simulink model "Question_1"  (R2024b)
settings: Solver=VariableStepAuto  StartTime=0.0  StopTime=10.0  RelTol=1e-3
model workspace (MAT data in the model file):
  b1 = 50
  b2 = 70
  k1 = 400
  k2 = 600
  m = 100
settings Model: Creator=Sagar  LastModifiedBy=Sagar

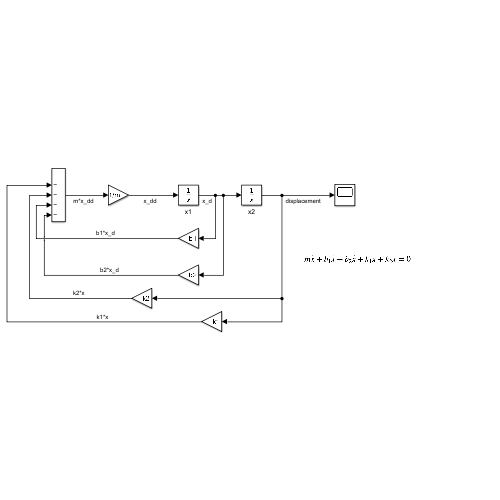
[thumbnail: Simulink's stored preview of the top-level diagram]
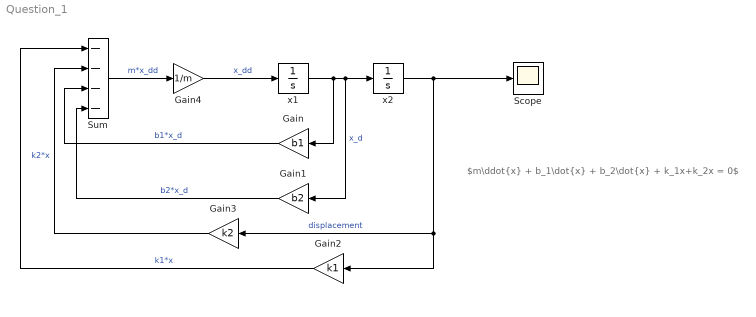
== system Question_1 ==
  note: $m\ddot{x} + b_1\dot{x} + b_2\dot{x} + k_1x+k_2x = 0$
  Gain : Gain  Gain=b1
  Gain1 : Gain  Gain=b2
  Gain2 : Gain  Gain=k1
  Gain3 : Gain  Gain=k2
  Gain4 : Gain  Gain=1/m
  Scope : Scope
  Sum : Sum  Inputs=|----
  x1 : Integrator
  x2 : Integrator  InitialCondition=0.8
  wires:
  Sum/1 -> Gain4/1  "m*x_dd"
  Gain4/1 -> x1/1  "x_dd"
  x1/1 -> Gain/1, Gain1/1, x2/1  "x_d"
  x2/1 -> Scope/1, Gain2/1, Gain3/1  "displacement"
  Gain/1 -> Sum/3  "b1*x_d"
  Gain1/1 -> Sum/4  "b2*x_d"
  Gain2/1 -> Sum/1  "k1*x"
  Gain3/1 -> Sum/2  "k2*x"
